simulink model "drawWorks_withLookup"  (R2018b)
settings: Solver=ode3  StartTime=0.0  StopTime=inf  RelTol=1e-3
PreLoadFcn:
  | addpath('CAD_Files');
  | warning('off','sm:sli:setup:compile:LocalSolverNotSupported');
  | 
  | loadScale = 3;
  | load limitsLookup.mat;
InitFcn:
  | Ts = 10e-4;        % SPS/Overall Simulation time step
  | Tssc = 10*Ts;       % Simscape simulation time step
  | 
  | G = 10;
  | Rdrum = 0.25;
  | Np = 5;
  | m_topdrive = 1000;
  | m_drillstring = 22500;
  | Rpulley = Rdrum;
  | 
  | m = m_topdrive + m_drillstring;
  | 
  | % Top/Bottom Distance
  | xtop = 48*0.3048;
  | xbott = 0;
  | 
  | % Maximum Torque/Power of Drive
  | Tmax = 8000*1.36;
  | Pmax = 1500*746;
  | 
  | % Initial Conditions
  | v0 = 0; %m/s
  | x0 = 0; %m
  | 
  | % Gravity
  | g = 9.8;
values from neighbouring files (symbols this model uses):
  distLowering = [-48 -47 -46 -45 -44 -43 -42 -41 -40 -39 -38 -37 ... (130 elements, 1x130)]    [limitsLookup.mat]
  distRaising = [0 0.1 0.2 0.3 0.4 0.5 0.6 0.7 0.8 0.9 1 1.1 ... (139 elements, 1x139)]    [limitsLookup.mat]
  loadIn = [23500 46000 68500 91000 93250 95500 97750 100000 102250 104500 106750 109000 ... (71 elements, 1x71)]    [DrawworksLimitData.mat]    (also in limitsLookup.mat)
  spdLowering = [-1500 -1500 -1500 -1500 -1500 -1500 -1500 -1500 -1500 -1500 -1483.12408278 -1433.71794393 ... (9230 elements, 71x130)]    [limitsLookup.mat]
  spdRaising = [7.42375457692 0 0 0 0 0 0 0 0 0 0 0 ... (9869 elements, 71x139)]    [limitsLookup.mat]
undefined symbols (not defined in the file or in its folder): DiscIntNeverNeededParam, X, Y, Z
libraries: sm_lib x38, fl_lib x14, nesl_utility x11, powerlib x6, simulink x6, spsDrivesDcBusModel x1
(part 2 of 2)

== system drawWorks_withLookup/Rig Frame/Pulley 1 ==
  Pulley Inertia : sm_lib/Body Elements/Solid  InertiaType=CalculateFromGeometry  Mass=0.01  MassUnits=kg  CenterOfMass=[0 0 0]  CenterOfMassUnits=m  MomentsOfInertia=[1 1 1]  MomentsOfInertiaUnits=kg*m^2  ProductsOfInertia=[0 0 0]  ProductsOfInertiaUnits=kg*m^2  BasedOnType=Density  Density=2700  DensityUnits=kg/m^3  DoExposeReferenceFrame=off  SerializedFrames=<Frames><Frame><Id>Frame1</Id><Value><Name>F1</Name><Origin><Source>GeometricFeature</Source><FeatureName>top surface</FeatureName></Origin><PrimaryAxis><DefinedDirection>+Z</DefinedDirection><Source>ReferenceFrame</Source><SourceDirection>+Z</SourceDirection><FeatureName></FeatureName></PrimaryAxis><SecondaryAxis><DefinedDirection>+X</DefinedDirection><Source>ReferenceFrame</Source><SourceDirection>+X</SourceDirection><FeatureName></FeatureName></SecondaryAxis></Value></Frame></Frames>  GraphicType=FromGeometry  MarkerShape=Frame  MarkerSize=10  GraphicVisPropType=SimpleVisualProperties  GraphicDiffuseColor=[1.0 1.0 1.0]  GraphicSpecularColor=[0.8 0.8 0.8]  GraphicAmbientColor=[0.15 0.15 0.15 1.0]  GraphicEmissiveColor=[0.0 0.0 0.0 1.0]  GraphicShininess=10  GraphicOpacity=1.0  GeometryShape=Cylinder  RectangleSize=[1 1]  RectangleSizeUnits=m  BrickDimensions=[1 1 1]  BrickDimensionUnits=m  CylinderRadius=Rpulley  CylinderRadiusUnits=m  CylinderLength=2  CylinderLengthUnits=in  SphereRadius=0.5  SphereRadiusUnits=in  EllipsoidRadii=[1 1 1]*0.1  EllipsoidRadiiUnits=m  ExtrusionCrossSection=[1 1; -1 1; -1 -1; 1 -1]  ExtrusionCrossSectionUnits=m  ExtrusionLength=1  ExtrusionLengthUnits=m  PolygonNumSides=3  PolygonOuterRadius=1  PolygonOuterRadiusUnits=m  ExtGeomFileType=STEP  ExtGeomFileName=winch.step  ExtGeomFileUnits=m  RevolutionCrossSection=[1 1; 1 -1; 2 -1; 2 1]  RevolutionCrossSectionUnits=m  RevolutionExtent=Full  RevolutionAngle=180  RevolutionAngleUnits=deg
  Revolute Joint : sm_lib/Joints/Revolute Joint  SenseConstraintForce=off  SenseConstraintForceX=off  SenseConstraintForceY=off  SenseConstraintForceZ=off  SenseConstraintTorque=off  SenseConstraintTorqueX=off  SenseConstraintTorqueY=off  SenseConstraintTorqueZ=off  SenseTotalForce=off  SenseTotalForceX=off  SenseTotalForceY=off  SenseTotalForceZ=off  SenseTotalTorque=off  SenseTotalTorqueX=off  SenseTotalTorqueY=off  SenseTotalTorqueZ=off  CompositeWrenchDir=FollowerOnBase  CompositeWrenchFrame=BaseFrame  EquilibriumPosition=0  EquilibriumPositionUnits=deg  SpringStiffness=0  SpringStiffnessUnits=N*m/deg  DampingCoefficient=0  DampingCoefficientUnits=N*m/(deg/s)  TorqueActuationMode=NoTorque  MotionActuationMode=ComputedMotion  SensePosition=off  SenseVelocity=off  SenseAcceleration=off  SenseTorqueForce=off  PositionTargetSpecify=off  PositionTargetPriority=High  PositionTargetValue=0  PositionTargetValueUnits=deg  VelocityTargetSpecify=off  VelocityTargetPriority=High  VelocityTargetValue=0  VelocityTargetValueUnits=deg/s
  Rigid Transform : sm_lib/Frames and Transforms/Rigid Transform  TranslationMethod=Cartesian  TranslationStandardOffset=0  TranslationLengthUnit=m  TranslationStandardAxis=+Z  TranslationCartesianOffset=[0 0 topOffset]  TranslationROffset=0  TranslationROffsetUnits=m  TranslationZOffset=0  TranslationZOffsetUnits=m  TranslationThetaOffset=0  TranslationThetaOffsetUnits=deg  RotationMethod=None  RotationAngleUnits=deg  RotationStandardAxis=+Z  RotationAngle=0.0  RotationArbitraryAxis=[0 0 1]  FollAlignAxisA=+X  BaseAlignAxisA=+Y  FollAlignAxisB=+Y  BaseAlignAxisB=+Z  RotationSequenceAxes=FollowerAxes  RotationSequence=XYX  RotationSequenceAngles=[0 0 0]  RotationSequenceAnglesUnits=deg  RotationMatrix=[1 0 0; 0 1 0; 0 0 1]
  Top : PMIOPort  Side=Left
  Pulley : PMIOPort  Port=2  Side=Right
  connections:
  Revolute Joint/RConn1 -- Pulley/RConn1 -- Pulley Inertia/LConn1
  Rigid Transform/RConn1 -- Revolute Joint/LConn1
  Top/RConn1 -- Rigid Transform/LConn1

== system drawWorks_withLookup/Rig Frame/Pulley 2 ==
  Pulley Inertia : sm_lib/Body Elements/Solid  InertiaType=CalculateFromGeometry  Mass=0.01  MassUnits=kg  CenterOfMass=[0 0 0]  CenterOfMassUnits=m  MomentsOfInertia=[1 1 1]  MomentsOfInertiaUnits=kg*m^2  ProductsOfInertia=[0 0 0]  ProductsOfInertiaUnits=kg*m^2  BasedOnType=Density  Density=2700  DensityUnits=kg/m^3  DoExposeReferenceFrame=off  SerializedFrames=<Frames><Frame><Id>Frame1</Id><Value><Name>F1</Name><Origin><Source>GeometricFeature</Source><FeatureName>top surface</FeatureName></Origin><PrimaryAxis><DefinedDirection>+Z</DefinedDirection><Source>ReferenceFrame</Source><SourceDirection>+Z</SourceDirection><FeatureName></FeatureName></PrimaryAxis><SecondaryAxis><DefinedDirection>+X</DefinedDirection><Source>ReferenceFrame</Source><SourceDirection>+X</SourceDirection><FeatureName></FeatureName></SecondaryAxis></Value></Frame></Frames>  GraphicType=FromGeometry  MarkerShape=Frame  MarkerSize=10  GraphicVisPropType=SimpleVisualProperties  GraphicDiffuseColor=[1.0 1.0 1.0]  GraphicSpecularColor=[0.8 0.8 0.8]  GraphicAmbientColor=[0.15 0.15 0.15 1.0]  GraphicEmissiveColor=[0.0 0.0 0.0 1.0]  GraphicShininess=10  GraphicOpacity=1.0  GeometryShape=Cylinder  RectangleSize=[1 1]  RectangleSizeUnits=m  BrickDimensions=[1 1 1]  BrickDimensionUnits=m  CylinderRadius=Rpulley  CylinderRadiusUnits=m  CylinderLength=2  CylinderLengthUnits=in  SphereRadius=0.5  SphereRadiusUnits=in  EllipsoidRadii=[1 1 1]*0.1  EllipsoidRadiiUnits=m  ExtrusionCrossSection=[1 1; -1 1; -1 -1; 1 -1]  ExtrusionCrossSectionUnits=m  ExtrusionLength=1  ExtrusionLengthUnits=m  PolygonNumSides=3  PolygonOuterRadius=1  PolygonOuterRadiusUnits=m  ExtGeomFileType=STEP  ExtGeomFileName=winch.step  ExtGeomFileUnits=m  RevolutionCrossSection=[1 1; 1 -1; 2 -1; 2 1]  RevolutionCrossSectionUnits=m  RevolutionExtent=Full  RevolutionAngle=180  RevolutionAngleUnits=deg
  Revolute Joint : sm_lib/Joints/Revolute Joint  SenseConstraintForce=off  SenseConstraintForceX=off  SenseConstraintForceY=off  SenseConstraintForceZ=off  SenseConstraintTorque=off  SenseConstraintTorqueX=off  SenseConstraintTorqueY=off  SenseConstraintTorqueZ=off  SenseTotalForce=off  SenseTotalForceX=off  SenseTotalForceY=off  SenseTotalForceZ=off  SenseTotalTorque=off  SenseTotalTorqueX=off  SenseTotalTorqueY=off  SenseTotalTorqueZ=off  CompositeWrenchDir=FollowerOnBase  CompositeWrenchFrame=BaseFrame  EquilibriumPosition=0  EquilibriumPositionUnits=deg  SpringStiffness=0  SpringStiffnessUnits=N*m/deg  DampingCoefficient=0  DampingCoefficientUnits=N*m/(deg/s)  TorqueActuationMode=NoTorque  MotionActuationMode=ComputedMotion  SensePosition=off  SenseVelocity=off  SenseAcceleration=off  SenseTorqueForce=off  PositionTargetSpecify=off  PositionTargetPriority=High  PositionTargetValue=0  PositionTargetValueUnits=deg  VelocityTargetSpecify=off  VelocityTargetPriority=High  VelocityTargetValue=0  VelocityTargetValueUnits=deg/s
  Rigid Transform : sm_lib/Frames and Transforms/Rigid Transform  TranslationMethod=Cartesian  TranslationStandardOffset=0  TranslationLengthUnit=m  TranslationStandardAxis=+Z  TranslationCartesianOffset=[0 0 topOffset]  TranslationROffset=0  TranslationROffsetUnits=m  TranslationZOffset=0  TranslationZOffsetUnits=m  TranslationThetaOffset=0  TranslationThetaOffsetUnits=deg  RotationMethod=None  RotationAngleUnits=deg  RotationStandardAxis=+Z  RotationAngle=0.0  RotationArbitraryAxis=[0 0 1]  FollAlignAxisA=+X  BaseAlignAxisA=+Y  FollAlignAxisB=+Y  BaseAlignAxisB=+Z  RotationSequenceAxes=FollowerAxes  RotationSequence=XYX  RotationSequenceAngles=[0 0 0]  RotationSequenceAnglesUnits=deg  RotationMatrix=[1 0 0; 0 1 0; 0 0 1]
  Top : PMIOPort  Side=Left
  Pulley : PMIOPort  Port=2  Side=Right
  connections:
  Pulley Inertia/LConn1 -- Revolute Joint/RConn1 -- Pulley/RConn1
  Rigid Transform/RConn1 -- Revolute Joint/LConn1
  Top/RConn1 -- Rigid Transform/LConn1

== system drawWorks_withLookup/Rig Frame/Pulley 3 ==
  Pulley Inertia : sm_lib/Body Elements/Solid  InertiaType=CalculateFromGeometry  Mass=0.01  MassUnits=kg  CenterOfMass=[0 0 0]  CenterOfMassUnits=m  MomentsOfInertia=[1 1 1]  MomentsOfInertiaUnits=kg*m^2  ProductsOfInertia=[0 0 0]  ProductsOfInertiaUnits=kg*m^2  BasedOnType=Density  Density=2700  DensityUnits=kg/m^3  DoExposeReferenceFrame=off  SerializedFrames=<Frames><Frame><Id>Frame1</Id><Value><Name>F1</Name><Origin><Source>GeometricFeature</Source><FeatureName>top surface</FeatureName></Origin><PrimaryAxis><DefinedDirection>+Z</DefinedDirection><Source>ReferenceFrame</Source><SourceDirection>+Z</SourceDirection><FeatureName></FeatureName></PrimaryAxis><SecondaryAxis><DefinedDirection>+X</DefinedDirection><Source>ReferenceFrame</Source><SourceDirection>+X</SourceDirection><FeatureName></FeatureName></SecondaryAxis></Value></Frame></Frames>  GraphicType=FromGeometry  MarkerShape=Frame  MarkerSize=10  GraphicVisPropType=SimpleVisualProperties  GraphicDiffuseColor=[1.0 1.0 1.0]  GraphicSpecularColor=[0.8 0.8 0.8]  GraphicAmbientColor=[0.15 0.15 0.15 1.0]  GraphicEmissiveColor=[0.0 0.0 0.0 1.0]  GraphicShininess=10  GraphicOpacity=1.0  GeometryShape=Cylinder  RectangleSize=[1 1]  RectangleSizeUnits=m  BrickDimensions=[1 1 1]  BrickDimensionUnits=m  CylinderRadius=Rpulley  CylinderRadiusUnits=m  CylinderLength=2  CylinderLengthUnits=in  SphereRadius=0.5  SphereRadiusUnits=in  EllipsoidRadii=[1 1 1]*0.1  EllipsoidRadiiUnits=m  ExtrusionCrossSection=[1 1; -1 1; -1 -1; 1 -1]  ExtrusionCrossSectionUnits=m  ExtrusionLength=1  ExtrusionLengthUnits=m  PolygonNumSides=3  PolygonOuterRadius=1  PolygonOuterRadiusUnits=m  ExtGeomFileType=STEP  ExtGeomFileName=winch.step  ExtGeomFileUnits=m  RevolutionCrossSection=[1 1; 1 -1; 2 -1; 2 1]  RevolutionCrossSectionUnits=m  RevolutionExtent=Full  RevolutionAngle=180  RevolutionAngleUnits=deg
  Revolute Joint : sm_lib/Joints/Revolute Joint  SenseConstraintForce=off  SenseConstraintForceX=off  SenseConstraintForceY=off  SenseConstraintForceZ=off  SenseConstraintTorque=off  SenseConstraintTorqueX=off  SenseConstraintTorqueY=off  SenseConstraintTorqueZ=off  SenseTotalForce=off  SenseTotalForceX=off  SenseTotalForceY=off  SenseTotalForceZ=off  SenseTotalTorque=off  SenseTotalTorqueX=off  SenseTotalTorqueY=off  SenseTotalTorqueZ=off  CompositeWrenchDir=FollowerOnBase  CompositeWrenchFrame=BaseFrame  EquilibriumPosition=0  EquilibriumPositionUnits=deg  SpringStiffness=0  SpringStiffnessUnits=N*m/deg  DampingCoefficient=0  DampingCoefficientUnits=N*m/(deg/s)  TorqueActuationMode=NoTorque  MotionActuationMode=ComputedMotion  SensePosition=off  SenseVelocity=off  SenseAcceleration=off  SenseTorqueForce=off  PositionTargetSpecify=off  PositionTargetPriority=High  PositionTargetValue=0  PositionTargetValueUnits=deg  VelocityTargetSpecify=off  VelocityTargetPriority=High  VelocityTargetValue=0  VelocityTargetValueUnits=deg/s
  Rigid Transform : sm_lib/Frames and Transforms/Rigid Transform  TranslationMethod=Cartesian  TranslationStandardOffset=0  TranslationLengthUnit=m  TranslationStandardAxis=+Z  TranslationCartesianOffset=[0 0 topOffset]  TranslationROffset=0  TranslationROffsetUnits=m  TranslationZOffset=0  TranslationZOffsetUnits=m  TranslationThetaOffset=0  TranslationThetaOffsetUnits=deg  RotationMethod=None  RotationAngleUnits=deg  RotationStandardAxis=+Z  RotationAngle=0.0  RotationArbitraryAxis=[0 0 1]  FollAlignAxisA=+X  BaseAlignAxisA=+Y  FollAlignAxisB=+Y  BaseAlignAxisB=+Z  RotationSequenceAxes=FollowerAxes  RotationSequence=XYX  RotationSequenceAngles=[0 0 0]  RotationSequenceAnglesUnits=deg  RotationMatrix=[1 0 0; 0 1 0; 0 0 1]
  Top : PMIOPort  Side=Left
  Pulley : PMIOPort  Port=2  Side=Right
  connections:
  Pulley Inertia/LConn1 -- Revolute Joint/RConn1 -- Pulley/RConn1
  Rigid Transform/RConn1 -- Revolute Joint/LConn1
  Top/RConn1 -- Rigid Transform/LConn1

== system drawWorks_withLookup/Shaft to Multibody/Rotational Simscape Intf ==
  Ideal Angular Velocity Source : fl_lib/Mechanical/Mechanical Sources/Ideal Angular Velocity Source
  Ideal Torque Sensor : fl_lib/Mechanical/Mechanical Sensors/Ideal Torque Sensor
  Mechanical Rotational Reference2 : fl_lib/Mechanical/Rotational Elements/Mechanical Rotational Reference
  w : PMIOPort  Side=Left
  t : PMIOPort  Port=2  Side=Right
  C : PMIOPort  Port=3  Side=Right
  connections:
  Ideal Angular Velocity Source/RConn1 -- w/RConn1
  Ideal Torque Sensor/RConn2 -- t/RConn1
  Ideal Angular Velocity Source/LConn1 -- Mechanical Rotational Reference2/LConn1
  Ideal Torque Sensor/RConn1 -- Ideal Angular Velocity Source/RConn2
  Ideal Torque Sensor/LConn1 -- C/RConn1

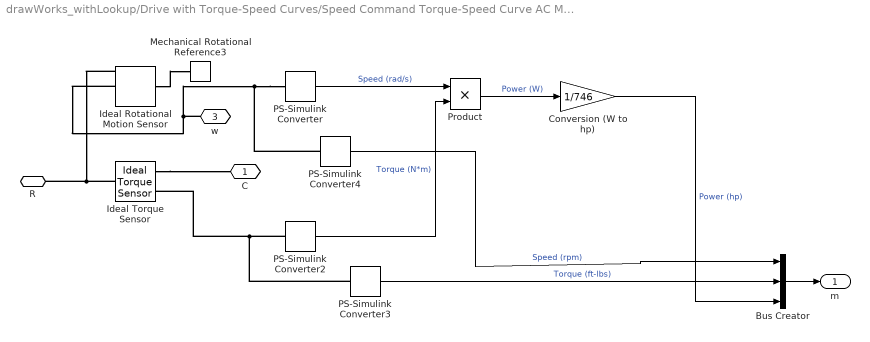
== system drawWorks_withLookup/Drive with Torque-Speed Curves/Speed Command Torque-Speed Curve AC Motor/Measurements ==
  Bus Creator : BusCreator  Inputs=3
  Conversion (W to hp) : Gain  Gain=1/746
  Ideal Rotational Motion Sensor : fl_lib/Mechanical/Mechanical Sensors/Ideal Rotational Motion Sensor  offset=0 rad
  Ideal Torque Sensor : fl_lib/Mechanical/Mechanical Sensors/Ideal Torque Sensor
  Mechanical Rotational Reference3 : fl_lib/Mechanical/Rotational Elements/Mechanical Rotational Reference
  PS-Simulink Converter : nesl_utility/PS-Simulink Converter  PhysicalDomain=network_engine_domain  SubClassName=ps_output  LeftPortType=input  RightPortType=output  PseudoPeriodic=off  Frequencies=[]  Unit=rad/s  AffineConversion=off
  PS-Simulink Converter2 : nesl_utility/PS-Simulink Converter  PhysicalDomain=network_engine_domain  SubClassName=ps_output  LeftPortType=input  RightPortType=output  PseudoPeriodic=off  Frequencies=[]  Unit=N*m  AffineConversion=off
  PS-Simulink Converter3 : nesl_utility/PS-Simulink Converter  PhysicalDomain=network_engine_domain  SubClassName=ps_output  LeftPortType=input  RightPortType=output  PseudoPeriodic=off  Frequencies=[]  Unit=lbf*ft  AffineConversion=off
  PS-Simulink Converter4 : nesl_utility/PS-Simulink Converter  PhysicalDomain=network_engine_domain  SubClassName=ps_output  LeftPortType=input  RightPortType=output  PseudoPeriodic=off  Frequencies=[]  Unit=rpm  AffineConversion=off
  Product : Product
  C : PMIOPort  Side=Right
  R : PMIOPort  Port=2  Side=Left
  w : PMIOPort  Port=3  Side=Right
  m : Outport
  wires:
  Bus Creator/1 -> m/1
  PS-Simulink Converter4/1 -> Bus Creator/1  "Speed (rpm)"
  PS-Simulink Converter3/1 -> Bus Creator/2  "Torque (ft-lbs)"
  Product/1 -> Conversion (W to hp)/1  "Power (W)"
  Conversion (W to hp)/1 -> Bus Creator/3  "Power (hp)"
  PS-Simulink Converter2/1 -> Product/2  "Torque (N*m)"
  PS-Simulink Converter/1 -> Product/1  "Speed (rad/s)"
  connections:
  Ideal Torque Sensor/RConn1 -- C/RConn1
  PS-Simulink Converter/LConn1 -- w/RConn1 -- Ideal Rotational Motion Sensor/RConn2 -- PS-Simulink Converter4/LConn1
  Ideal Torque Sensor/RConn2 -- PS-Simulink Converter3/LConn1 -- PS-Simulink Converter2/LConn1
  Ideal Torque Sensor/LConn1 -- Ideal Rotational Motion Sensor/RConn1 -- R/RConn1
  Ideal Rotational Motion Sensor/LConn1 -- Mechanical Rotational Reference3/LConn1

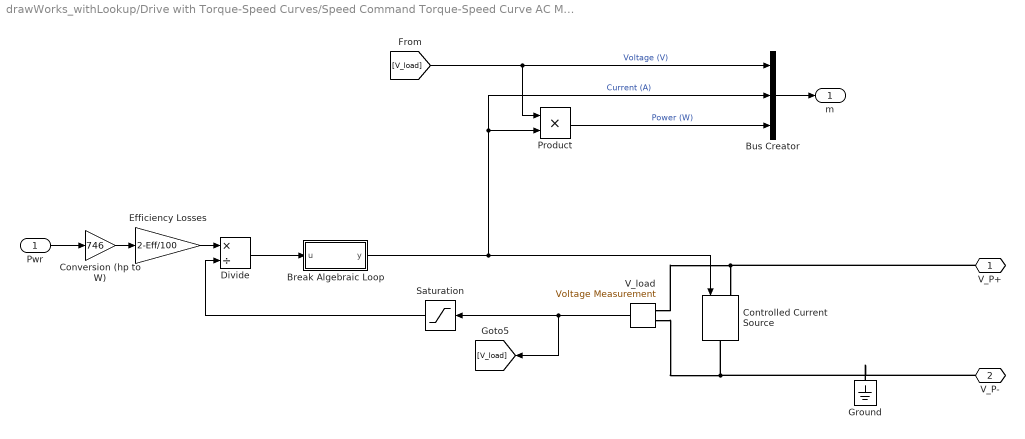
== system drawWorks_withLookup/Drive with Torque-Speed Curves/Speed Command Torque-Speed Curve AC Motor/Power Load ==
  Pwr : Inport
  Break Algebraic Loop : Subsystem
  Bus Creator : BusCreator  Inputs=3
  Controlled Current Source : powerlib/Electrical Sources/Controlled Current Source  Initialize=off  Source_Type=AC  Amplitude=0  Phase=0  Frequency=0  Measurements=None
  Conversion (hp to W) : Gain  Gain=746
  Divide : Product  Inputs=*/
  Efficiency Losses : Gain  Gain=2-Eff/100
  Ground : powerlib/Elements/Ground  LConnTagsString=a
  Product : Product
  Saturation : Saturate  UpperLimit=inf  LowerLimit=1e-3
  V_load : powerlib/Measurements/Voltage Measurement  PhasorSimulation=off  OutputType=Complex  PSBequivalent=0
  V_P+ : PMIOPort  Side=Left
  V_P- : PMIOPort  Port=2  Side=Left
  m : Outport
  wires:
  V_load/1 -> [V_load], Saturation/1
  Divide/1 -> Break Algebraic Loop/1(u)
  Bus Creator/1 -> m/1
  Product/1 -> Bus Creator/3  "Power (W)"
  Saturation/1 -> Divide/2
  Break Algebraic Loop/1(y) -> Controlled Current Source/1, Bus Creator/2, Product/2  "Current (A)"
  [V_load] -> Product/1, Bus Creator/1  "Voltage (V)"
  Pwr/1 -> Conversion (hp to W)/1
  Conversion (hp to W)/1 -> Efficiency Losses/1
  Efficiency Losses/1 -> Divide/1
  connections:
  V_load/LConn2 -- V_P-/RConn1 -- Ground/LConn1 -- Controlled Current Source/RConn1
  V_load/LConn1 -- V_P+/RConn1 -- Controlled Current Source/LConn1

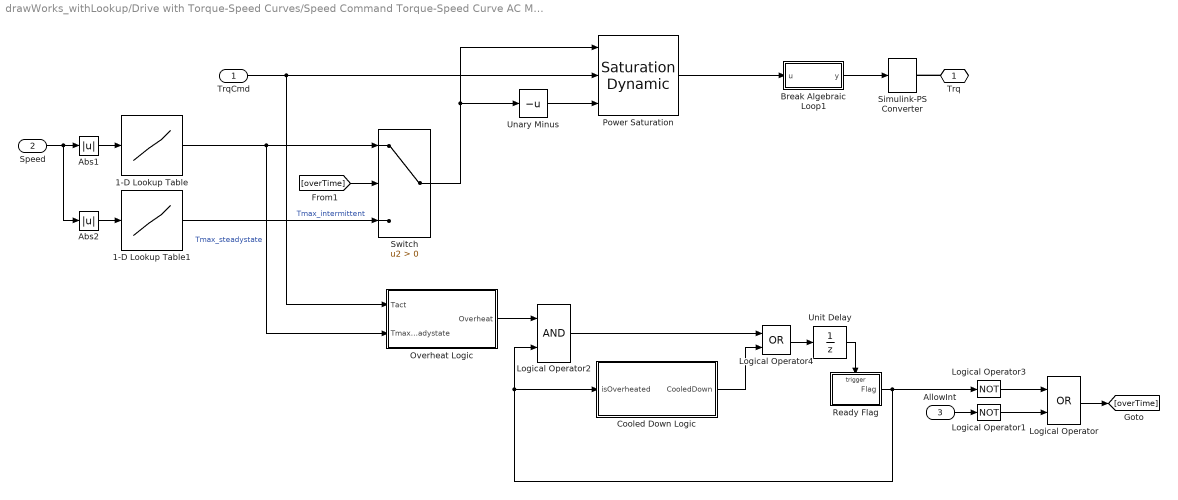
== system drawWorks_withLookup/Drive with Torque-Speed Curves/Speed Command Torque-Speed Curve AC Motor/Torque-Speed Curve ==
  TrqCmd : Inport
  Speed : Inport  Port=2
  AllowInt : Inport  Port=3
  1-D Lookup Table : Lookup_n-D  NumberOfTableDimensions=1  BreakpointsForDimension1=contSpd  Table=contTrq  InternalRulePriority=Speed  RndMeth=Simplest  InputSameDT=on
  1-D Lookup Table1 : Lookup_n-D  NumberOfTableDimensions=1  BreakpointsForDimension1=intSpd  Table=intTrq  InternalRulePriority=Speed  RndMeth=Simplest  InputSameDT=on
  Abs1 : Abs
  Abs2 : Abs
  Break Algebraic Loop1 : Subsystem
  Cooled Down Logic : Subsystem
  Logical Operator : Logic  Operator=OR  AllPortsSameDT=off  OutDataTypeStr=boolean
  Logical Operator1 : Logic  Operator=NOT  AllPortsSameDT=off  OutDataTypeStr=boolean
  Logical Operator2 : Logic  AllPortsSameDT=off  OutDataTypeStr=boolean
  Logical Operator3 : Logic  Operator=NOT  AllPortsSameDT=off  OutDataTypeStr=boolean
  Logical Operator4 : Logic  Operator=OR  AllPortsSameDT=off  OutDataTypeStr=boolean
  Overheat Logic : Subsystem
  Power Saturation : simulink/Discontinuities/Saturation Dynamic  OutMin=[]  OutMax=[]  OutDataTypeStr=Inherit: Same as second input  OutDataType=fixdt(1, 16)  OutScaling=2^-10  DoSatur=off
  Ready Flag : Subsystem  TreatAsAtomicUnit=on
  Simulink-PS Converter : nesl_utility/Simulink-PS Converter  PhysicalDomain=network_engine_domain  SubClassName=ps_input  LeftPortType=input  RightPortType=output  PseudoPeriodic=off  Frequencies=[]  NoiseDistribution=none  NoiseParameters=[]  Unit=ft*lb  AffineConversion=off  FilteringAndDerivatives=provide  SimscapeFilterOrder=2  InputFilterTimeConstant=0.001  UdotUserProvided=0
  Switch : Switch  Criteria=u2 > Threshold
  Unary Minus : UnaryMinus
  Unit Delay : UnitDelay  SampleTime=Tssc
  Trq : PMIOPort  Side=Right
  wires:
  Cooled Down Logic/1(CooledDown) -> Logical Operator4/2
  Logical Operator/1 -> [overTime]
  Overheat Logic/1(Overheat) -> Logical Operator2/1
  Unit Delay/1 -> Ready Flag/Trigger
  1-D Lookup Table/1 -> Switch/1, Overheat Logic/2(Tmax_steadystate)  "Tmax_steadystate"
  Speed/1 -> Abs2/1, Abs1/1
  Unary Minus/1 -> Power Saturation/3
  Switch/1 -> Unary Minus/1, Power Saturation/1
  Power Saturation/1 -> Break Algebraic Loop1/1(u)
  Logical Operator3/1 -> Logical Operator/1
  Logical Operator1/1 -> Logical Operator/2
  Ready Flag/1(Flag) -> Logical Operator2/2, Cooled Down Logic/1(isOverheated), Logical Operator3/1
  Logical Operator2/1 -> Logical Operator4/1
  Logical Operator4/1 -> Unit Delay/1
  [overTime] -> Switch/2
  1-D Lookup Table1/1 -> Switch/3  "Tmax_intermittent"
  TrqCmd/1 -> Overheat Logic/1(Tact), Power Saturation/2
  Abs1/1 -> 1-D Lookup Table/1
  Abs2/1 -> 1-D Lookup Table1/1
  AllowInt/1 -> Logical Operator1/1
  Break Algebraic Loop1/1(y) -> Simulink-PS Converter/1
  connections:
  Trq/RConn1 -- Simulink-PS Converter/RConn1

== system drawWorks_withLookup/Drive with Torque-Speed Curves/Speed Command Torque-Speed Curve AC Motor/Power Load/Break Algebraic Loop ==
  u : Inport
  1/T : Gain  Gain=1/T_alg
  Discrete-Time Integrator : DiscreteIntegrator  SampleTime=-1  ICPrevOutput=DiscIntNeverNeededParam  ICPrevScaledInput=DiscIntNeverNeededParam
  Sum : Sum  Inputs=|+-
  y : Outport
  wires:
  Sum/1 -> 1/T/1
  Discrete-Time Integrator/1 -> y/1, Sum/2
  1/T/1 -> Discrete-Time Integrator/1
  u/1 -> Sum/1

== system drawWorks_withLookup/Drive with Torque-Speed Curves/Speed Command Torque-Speed Curve AC Motor/Torque-Speed Curve/Break Algebraic Loop1 ==
  u : Inport
  1/T : Gain  Gain=1/T_alg
  Discrete-Time Integrator : DiscreteIntegrator  InitialCondition=Rdrum/(G*(Np-1))*(m_topdrive+m_drillstring)*9.81*0.737562*loadScale  SampleTime=-1  ICPrevOutput=DiscIntNeverNeededParam  ICPrevScaledInput=DiscIntNeverNeededParam
  Sum : Sum  Inputs=|+-
  y : Outport
  wires:
  Sum/1 -> 1/T/1
  Discrete-Time Integrator/1 -> y/1, Sum/2
  1/T/1 -> Discrete-Time Integrator/1
  u/1 -> Sum/1

== system drawWorks_withLookup/Drive with Torque-Speed Curves/Speed Command Torque-Speed Curve AC Motor/Torque-Speed Curve/Cooled Down Logic ==
  isOverheated : Inport
  Compare To Constant1 : simulink/Logic and Bit Operations/Compare To Constant  relop=>=  const=offTime  OutDataTypeStr=boolean
  Logical Operator3 : Logic  AllPortsSameDT=off  OutDataTypeStr=boolean
  Logical Operator5 : Logic  Operator=NOT  AllPortsSameDT=off  OutDataTypeStr=boolean
  Measure Time In Steady State : Subsystem
  CooledDown : Outport
  wires:
  isOverheated/1 -> Logical Operator5/1
  Compare To Constant1/1 -> Logical Operator3/1
  Logical Operator3/1 -> CooledDown/1
  Logical Operator5/1 -> Logical Operator3/2, Measure Time In Steady State/1(In Steady State)
  Measure Time In Steady State/1(Time Elapse) -> Compare To Constant1/1

== system drawWorks_withLookup/Drive with Torque-Speed Curves/Speed Command Torque-Speed Curve AC Motor/Torque-Speed Curve/Overheat Logic ==
  Tact : Inport
  Tmax_steadystate : Inport  Port=2
  Abs4 : Abs
  Compare To Constant : simulink/Logic and Bit Operations/Compare To Constant  relop=>=  const=intTime  OutDataTypeStr=boolean
  Measure Time Above Steady State : Subsystem
  Relational Operator : RelationalOperator  OutDataTypeStr=boolean  RndMeth=Simplest
  Overheat : Outport
  wires:
  Tmax_steadystate/1 -> Relational Operator/2
  Relational Operator/1 -> Measure Time Above Steady State/1(In Intermittent)
  Abs4/1 -> Relational Operator/1
  Tact/1 -> Abs4/1
  Measure Time Above Steady State/1(Time Elapse) -> Compare To Constant/1
  Compare To Constant/1 -> Overheat/1

== system drawWorks_withLookup/Drive with Torque-Speed Curves/Speed Command Torque-Speed Curve AC Motor/Torque-Speed Curve/Ready Flag ==
  Trigger : TriggerPort  VariantControl=Variant
  Repeating Sequence Stair : simulink/Sources/Repeating Sequence Stair  OutValues=[0 1]  tsamp=-1  OutMin=[]  OutMax=[]  OutDataTypeStr=double  OutputDataTypeScalingMode=double  OutDataType=fixdt(0,8)  ConRadixGroup=Best Precision: Vector-wise  OutScaling=2^-12
  Flag : Outport  InitialOutput=1
  wires:
  Repeating Sequence Stair/1 -> Flag/1

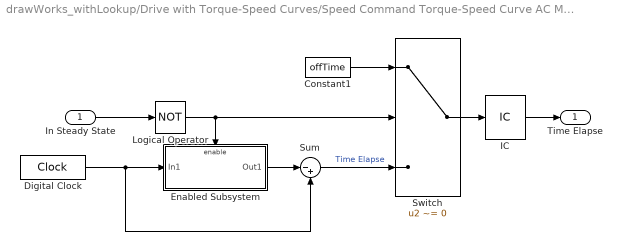
== system drawWorks_withLookup/Drive with Torque-Speed Curves/Speed Command Torque-Speed Curve AC Motor/Torque-Speed Curve/Cooled Down Logic/Measure Time In Steady State ==
  In Steady State : Inport
  Constant1 : Constant  Value=offTime
  Digital Clock : DigitalClock  SampleTime=Tssc
  Enabled Subsystem : Subsystem  TreatAsAtomicUnit=on
  IC : InitialCondition  Value=offTime
  Logical Operator : Logic  Operator=NOT  AllPortsSameDT=off  OutDataTypeStr=boolean
  Sum : Sum  Inputs=|-+
  Switch : Switch  Criteria=u2 ~= 0
  Time Elapse : Outport
  wires:
  IC/1 -> Time Elapse/1
  Switch/1 -> IC/1
  Constant1/1 -> Switch/1
  Logical Operator/1 -> Switch/2, Enabled Subsystem/Enable
  In Steady State/1 -> Logical Operator/1
  Digital Clock/1 -> Sum/2, Enabled Subsystem/1(In1)
  Sum/1 -> Switch/3  "Time Elapse"
  Enabled Subsystem/1(Out1) -> Sum/1

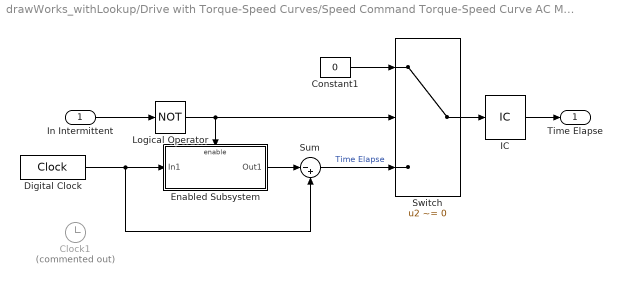
== system drawWorks_withLookup/Drive with Torque-Speed Curves/Speed Command Torque-Speed Curve AC Motor/Torque-Speed Curve/Overheat Logic/Measure Time Above Steady State ==
  In Intermittent : Inport
  Clock1 : Clock  Commented=on
  Constant1 : Constant  Value=0
  Digital Clock : DigitalClock  SampleTime=Tssc
  Enabled Subsystem : Subsystem  TreatAsAtomicUnit=on
  IC : InitialCondition  Value=0
  Logical Operator : Logic  Operator=NOT  AllPortsSameDT=off  OutDataTypeStr=boolean
  Sum : Sum  Inputs=|-+
  Switch : Switch  Criteria=u2 ~= 0
  Time Elapse : Outport
  wires:
  Enabled Subsystem/1(Out1) -> Sum/1
  Sum/1 -> Switch/3  "Time Elapse"
  Digital Clock/1 -> Enabled Subsystem/1(In1), Sum/2
  In Intermittent/1 -> Logical Operator/1
  Logical Operator/1 -> Enabled Subsystem/Enable, Switch/2
  Constant1/1 -> Switch/1
  Switch/1 -> IC/1
  IC/1 -> Time Elapse/1

== system drawWorks_withLookup/Drive with Torque-Speed Curves/Speed Command Torque-Speed Curve AC Motor/Torque-Speed Curve/Cooled Down Logic/Measure Time In Steady State/Enabled Subsystem ==
  In1 : Inport
  Enable : EnablePort
  Out1 : Outport
  wires:
  In1/1 -> Out1/1

== system drawWorks_withLookup/Drive with Torque-Speed Curves/Speed Command Torque-Speed Curve AC Motor/Torque-Speed Curve/Overheat Logic/Measure Time Above Steady State/Enabled Subsystem ==
  In1 : Inport
  Enable : EnablePort
  Out1 : Outport
  wires:
  In1/1 -> Out1/1

== stateflow chart drawWorks_withLookup/Lookup Limit Logic and Auto-Driller ==
  state Manual
    [wout,wlimit] = EnergySpeedLimiter(wcmd,m,x);
  state AutoDriller
    state InitalizeAuto
    state RaiseHoist
      [wout,wlimit] = EnergySpeedLimiter(1500,m,x);
    state AddPipeAndMake
      wout = 0;
    state LowerAndDrill
      [wout,wlimit] = EnergySpeedLimiter(-1500,m,x);
    state BreakString
      wout = 0;
    (default) -> InitalizeAuto
    InitalizeAuto -> RaiseHoist : [after(2,sec)]
    BreakString -> RaiseHoist : [after(5,sec)]
    RaiseHoist -> AddPipeAndMake : [x >= xtop*0.995]
    AddPipeAndMake -> LowerAndDrill : [after(5,sec)]
    LowerAndDrill -> BreakString : [x <= 0.01]
  state DisableLimits
    wout = wcmd;
    wlimit = [2000;-2000];
  state [wout,wlimits] = EnergySpeedLimiter(wcmd,m,x) [function]
  (default) -> Manual
  Manual -> AutoDriller [order 2] : [autoDriller == 1]
  AutoDriller -> Manual : [autoDriller == 0]
  Manual -> DisableLimits [order 1] : [disableLimit == 1]
  DisableLimits -> Manual : [disableLimit == 0]
  data: wcmd function_input double size=1; m function_input double size=1; x function_input double size=1; wout function_output; wlimits function_output; wcmd input double size=1; x input double size=1; m input double size=1; disableLimit input boolean size=1; autoDriller input boolean size=1; wout output double size=1; xtop constant double =48; wlimit output double size=2
